simulink model "es2_sim"  (Simulink 7.5)
settings: Solver=ode45  StartTime=0.0  StopTime=10.0  RelTol=1e-3
libraries: simulink x1
settings Model: Creator=76936  LastModifiedBy=76936

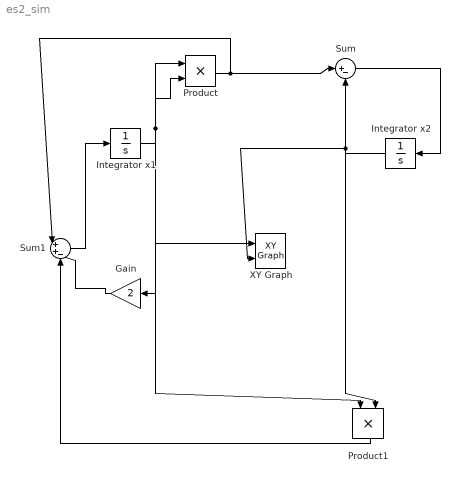
== system es2_sim ==
  Gain : Gain  Gain=2  ParameterDataType=fixdt(1, 16)  ParameterScaling=2^0  OutDataType=fixdt(1, 16)  OutScaling=2^0
  Integrator x1 : Integrator  InitialCondition=-1
  Integrator x2 : Integrator  InitialCondition=-1
  Product : Product  OutDataType=fixdt(1, 16)  OutScaling=2^0  RndMeth=Zero
  Product1 : Product  OutDataType=fixdt(1, 16)  OutScaling=2^0  RndMeth=Zero
  Sum : Sum  Inputs=|+-  OutDataType=fixdt(1, 16)  OutScaling=2^0
  Sum1 : Sum  Inputs=|++-  OutDataType=fixdt(1, 16)  OutScaling=2^0
  XY Graph : simulink/Sinks/XY Graph  SystemSampleTime=-1  xmin=-5  xmax=5  ymin=-5  ymax=5  st=-1
  wires:
  Integrator x1/1 -> Product/2, Product/1, Gain/1, Product1/1, XY Graph/1
  Product/1 -> Sum/1, Sum1/1
  Integrator x2/1 -> Sum/2, Product1/2, XY Graph/2
  Sum/1 -> Integrator x2/1
  Gain/1 -> Sum1/2
  Product1/1 -> Sum1/3
  Sum1/1 -> Integrator x1/1
